simulink model "Simulink_Ruido"  (R2020b)
settings: Solver=VariableStepAuto  StartTime=0.0  StopTime=50  RelTol=1e-3
model workspace (MAT data in the model file):
  Upsample = 5
libraries: dspfdesign x3, commchan3 x2, dspsrcs4 x2, dspsnks4 x1, dspvision x1, dspsigops x1
settings Model: Creator=enrique  LastModifiedBy=enrique

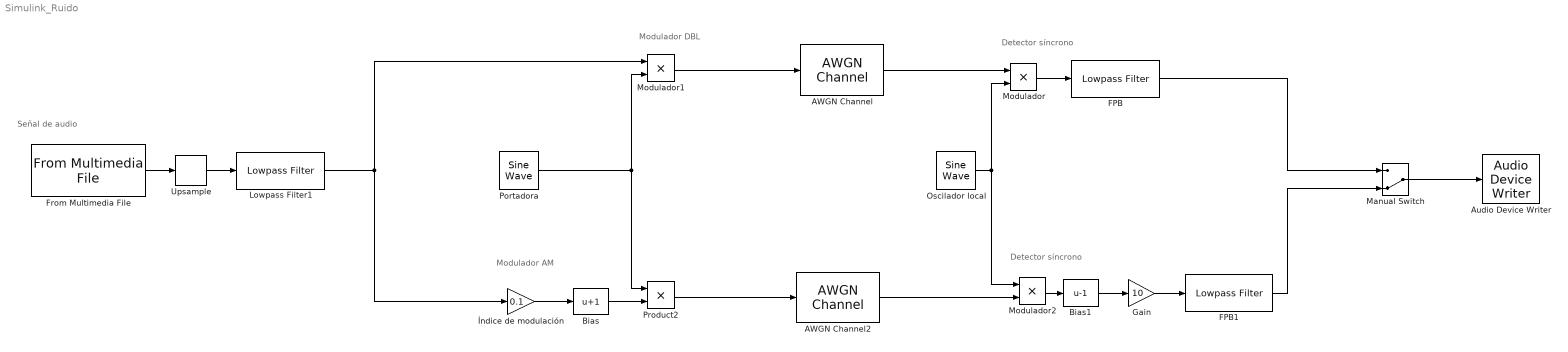
== system Simulink_Ruido ==
  note: Modulador DBL
  note: Detector síncrono
  note: Señal de audio
  note: Modulador AM
  note: Detector síncrono
  AWGN Channel : commchan3/AWGN Channel  InputProcessing=Columns as channels (frame based)  seed=67  noiseMode="Signal to noise ratio  (SNR)"  EbNodB=10  EsNodB=10  SNRdB=20  bitsPerSym=1  Ps=.25  Tsym=1  variance=1
  AWGN Channel2 : commchan3/AWGN Channel  InputProcessing=Columns as channels (frame based)  seed=67  noiseMode="Signal to noise ratio  (SNR)"  EbNodB=10  EsNodB=10  SNRdB=20  bitsPerSym=1  Ps=.25  Tsym=1  variance=1
  Audio Device Writer : dspsnks4/Audio Device Writer  Driver=CoreAudio  Device=Salida integrada  InheritSampleRate=on  SampleRate=44100  BitDepth=16-bit integer  BufferSize=4096  NumBuffers=10  DefaultOutputChannelMapping=on  OutputChannelMapping=1:2  OutputNumUnderrunSamples=off  DriverIdx=5  DeviceWarnFlag=''
  Bias : Bias  Bias=1
  Bias1 : Bias  Bias=-1
  FPB : dspfdesign/Lowpass Filter  FilterType=FIR  DesignForMinimumOrder=on  FilterOrder=50  PassbandFrequency=12000  StopbandFrequency=15000  PassbandRipple=0.1  StopbandAttenuation=80  InheritSampleRate=off  SampleRate=5*22050  SimulateUsing=Interpreted execution  roundingMode=Floor  coeffsDataTypeStr=fixdt(1,16)
  FPB1 : dspfdesign/Lowpass Filter  FilterType=FIR  DesignForMinimumOrder=on  FilterOrder=50  PassbandFrequency=12000  StopbandFrequency=15000  PassbandRipple=0.1  StopbandAttenuation=80  InheritSampleRate=off  SampleRate=5*22050  SimulateUsing=Interpreted execution  roundingMode=Floor  coeffsDataTypeStr=fixdt(1,16)
  From Multimedia File : dspvision/From Multimedia File  inputFilename=speech_dft.mp3  readRange=[1 Inf]  loop=on  numPlays=Inf  outputStreams=Audio only  videoDataType=single  audioDataType=double  inheritSampleTime=on  userDefinedSampleTime=1/30  noAudioOutput=off  isIntensityVideo=off  fourcc=RGB  colorVideoFormat=Separate color signals  outputEOF=off  dataOrg=Column-major  audioFrameSize=1024  computeAudioFrameSize=off  outSamplingMode=Sample based
  Gain : Gain  Gain=10
  Lowpass Filter1 : dspfdesign/Lowpass Filter  FilterType=FIR  DesignForMinimumOrder=on  FilterOrder=50  PassbandFrequency=12e3  StopbandFrequency=15e3  PassbandRipple=0.1  StopbandAttenuation=80  InheritSampleRate=off  SampleRate=5*22050  SimulateUsing=Interpreted execution  roundingMode=Floor  coeffsDataTypeStr=fixdt(1,16)
  Manual Switch : ManualSwitch  CurrentSetting=0
  Modulador : Product  OutDataTypeStr=Inherit: Same as first input
  Modulador1 : Product  OutDataTypeStr=Inherit: Same as first input
  Modulador2 : Product  OutDataTypeStr=Inherit: Same as first input
  Oscilador local : dspsrcs4/Sine Wave  Amplitude=2  Frequency=30000  Phase=0  SampleMode=Discrete  OutComplex=Real  CompMethod=Trigonometric fcn  TableSize=Speed  SampleTime=1/(22050*5)  SamplesPerFrame=1024*5  ResetState=Catch up to simulation time  OutputFrames=off  dataType=double  wordLen=16  udDataType=sfix(16)  fracBitsMode=Best precision  numFracBits=15  OutDataTypeStr=double  LastOutDataTypeStr=double
  Portadora : dspsrcs4/Sine Wave  Amplitude=1  Frequency=30000  Phase=0  SampleMode=Discrete  OutComplex=Real  CompMethod=Trigonometric fcn  TableSize=Speed  SampleTime=1/(22050*5)  SamplesPerFrame=1024*5  ResetState=Catch up to simulation time  OutputFrames=off  dataType=double  wordLen=16  udDataType=sfix(16)  fracBitsMode=Best precision  numFracBits=15  OutDataTypeStr=double  LastOutDataTypeStr=double
  Product2 : Product  OutDataTypeStr=Inherit: Same as first input
  Upsample : dspsigops/Upsample  N=5  phase=0  InputProcessing=Columns as channels (frame based)  RateOptions=Enforce single-rate processing  ic=0  mode=Unused parameter value
  "Índice de modulación " : Gain  Gain=0.1
  wires:
  From Multimedia File/1 -> Upsample/1
  Upsample/1 -> Lowpass Filter1/1
  Oscilador local/1 -> Modulador/2, Modulador2/1
  Modulador/1 -> FPB/1
  Modulador1/1 -> AWGN Channel/1
  AWGN Channel/1 -> Modulador/1
  "Índice de modulación "/1 -> Bias/1
  Bias/1 -> Product2/2
  Lowpass Filter1/1 -> Modulador1/1, "Índice de modulación "/1
  Portadora/1 -> Modulador1/2, Product2/1
  Product2/1 -> AWGN Channel2/1
  Manual Switch/1 -> Audio Device Writer/1
  FPB/1 -> Manual Switch/1
  FPB1/1 -> Manual Switch/2
  Modulador2/1 -> Bias1/1
  Bias1/1 -> Gain/1
  Gain/1 -> FPB1/1
  AWGN Channel2/1 -> Modulador2/2
